simulink model "battery_sim"  (R2022a)
settings: Solver=VariableStepAuto  StartTime=0.0  StopTime=4000  RelTol=1e-3
undefined symbols (not defined in the file): T_AMB
libraries: fl_lib x13, nesl_utility x1
settings Model: DataDictionary=battery.sldd  Creator=Cristobal  LastModifiedBy=Cristobal
settings SFSimCC: SimTargetLang=C++  GPUAcceleration=on  SimDLTargetLibrary=cudnn

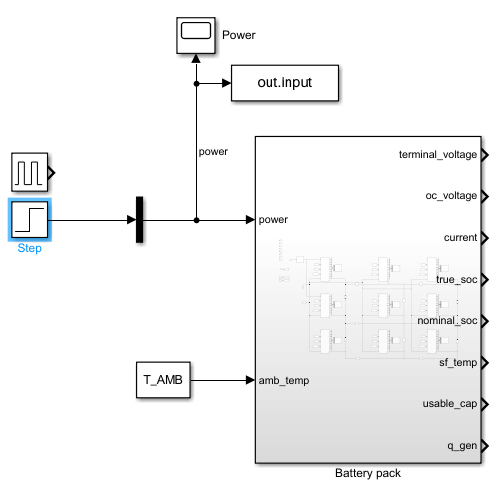
[thumbnail: Simulink's stored preview of the top-level diagram]
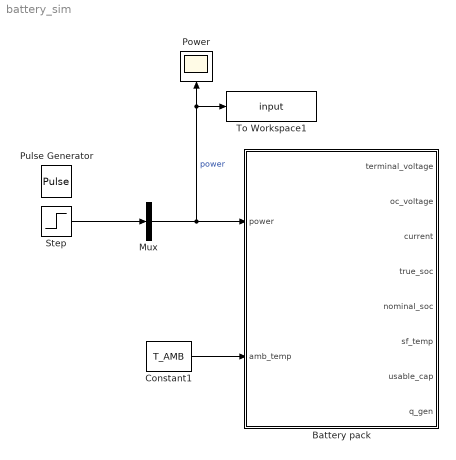
== system battery_sim ==
  Battery pack : Subsystem
  Constant1 : Constant  Value=T_AMB
  Mux : Mux  Inputs=1
  Power : Scope
  Pulse Generator : DiscretePulseGenerator  PulseType=Time based  Amplitude=1e-1  Period=300  PulseWidth=50
  Step : Step  Time=0  After=80  SampleTime=0
  To Workspace1 : ToWorkspace  VariableName=input  SaveFormat=Timeseries  SampleTime=-1
  wires:
  Constant1/1 -> Battery pack/2(amb_temp)
  Mux/1 -> To Workspace1/1, Power/1, Battery pack/1(power)  "power"
  Step/1 -> Mux/1

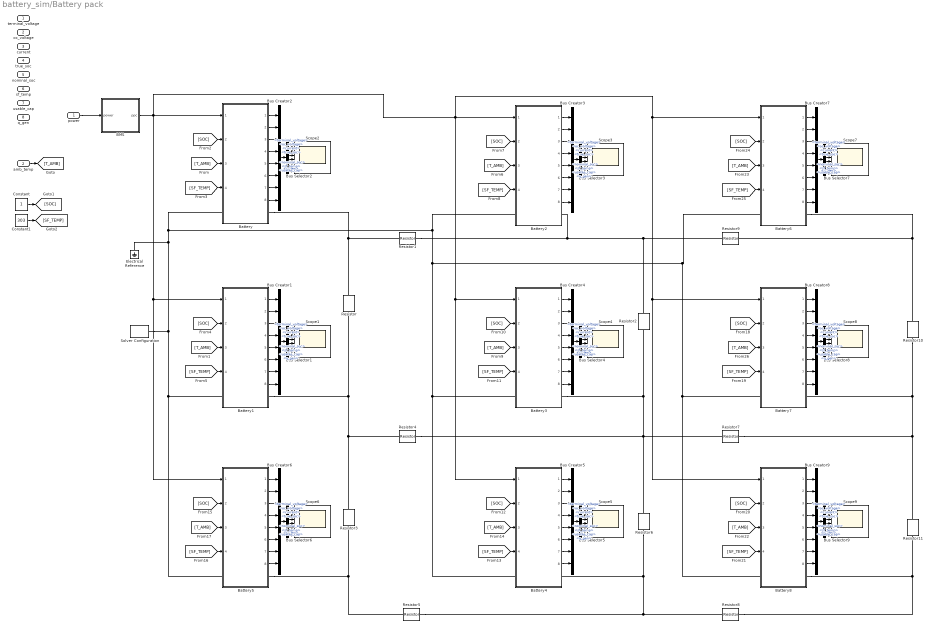
== system battery_sim/Battery pack ==
  power : Inport
  amb_temp : Inport  Port=2
  BMS : Subsystem  mask{Outputs=9}
      mask init:
      | % for i = 1:Outputs
      |     %     replace_block(gcb, "Name", "Terminator" + i, "Outport", "noprompt");
      |     % end
      |     % for i = Outputs + 1:64
      |     %     replace_block(gcb, "Name", "Terminator" + i, "Terminator", "noprompt");
      |     % end
      mask DialogControl DescGroupVar Prompt: BMS
      mask DialogControl DescTextVar Prompt: Ideal BMS that evenly distributes power
  Battery{,1..8} (9 alike) : Subsystem  ReferencedSubsystem=battery
  Bus Creator{1..9} (9 alike) : BusCreator  Inputs=8
  Bus Selector{1..9} (9 alike) : BusSelector  OutputSignals=terminal_voltage,oc_voltage,current,true_soc,nominal_soc,sf_temp,usable_cap,q_gen
  Constant : Constant
  Constant1 : Constant  Value=303
  Electrical Reference : fl_lib/Electrical/Electrical Elements/Electrical Reference
      settings: SourceProductBaseCode=PW,SS,VE
  Resistor{,1..11} (12 alike) : fl_lib/Electrical/Electrical Elements/Resistor  R=1e12 Ohm  i_specify=off  i_priority=None  i=0 A  i_nominal_specify=off  i_nominal_unit=A  i_nominal_value=1  v_specify=off  v_priority=None  v=0 V  v_nominal_specify=off  v_nominal_unit=V  v_nominal_value=1
      settings: SourceProductBaseCode=PW,SS,VE
  Scope{1..9} (9 alike) : Scope  NumInputPorts=8
  Solver Configuration : nesl_utility/Solver Configuration  PhysicalDomain=network_engine_domain  SubClassName=solver  LeftPortType=input  RightPortType=generic  Tones=[]  Harmonics=[]  SimulateNoise=off  Profile=off  UseLocalSampling=off  EnableSwitchedLinearOptims=on  FrequencyDomain=off  UseCCode=off  RelTol=0.001  AbsTol=0.001  MinStep=1e-09  ToWorkspace=off  RevertToSquareIcSolve=off  NumHomotopyIterations=100  PhasorMode=off  PhasorModeNumHarmonics=1  IndexReductionMethod=DerivativeReplacement  DoDC=off  ResidualTolerance=1e-09  UseLocalSolver=off  LocalSolverChoice=NE_BACKWARD_EULER_ADVANCER  LocalSolverSampleTime=0.001  DoFixedCost=off  MaxNonlinIter=3  MaxModeIter=2  ComputeImpulses=off  ImpulseIterations=2  LinearAlgebra=auto  LinearAlgebraNumThread=0  EquationFormulation=NE_TIME_EF  DelaysMemoryBudget=1024  AutomaticFiltering=on  FilteringTimeConstant=0.001  PartitionStorageMethod=AS_NEEDED  PartitionMemoryBudget=1024  PartitionMethod=ROBUST
      settings: SourceProductBaseCode=SS,PW,VE
  terminal_voltage : Outport
  oc_voltage : Outport  Port=2
  current : Outport  Port=3
  true_soc : Outport  Port=4
  nominal_soc : Outport  Port=5
  sf_temp : Outport  Port=6
  usable_cap : Outport  Port=7
  q_gen : Outport  Port=8
  wires:
  Bus Selector1/1 -> Scope1/1  "<terminal_voltage>"
  Bus Selector1/6 -> Scope1/6  "<sf_temp>"
  Bus Selector1/7 -> Scope1/7  "<usable_cap>"
  Bus Selector1/3 -> Scope1/3  "<current>"
  Bus Selector1/5 -> Scope1/5  "<nominal_soc>"
  Bus Selector1/2 -> Scope1/2  "<oc_voltage>"
  Bus Selector1/4 -> Scope1/4  "<true_soc>"
  Bus Selector1/8 -> Scope1/8  "<q_gen>"
  Battery1/1 -> Bus Creator1/1
  Battery1/2 -> Bus Creator1/2
  Battery1/3 -> Bus Creator1/3
  Battery1/4 -> Bus Creator1/4
  Battery1/5 -> Bus Creator1/5
  Battery1/6 -> Bus Creator1/6
  Battery1/7 -> Bus Creator1/7
  Battery1/8 -> Bus Creator1/8
  Bus Creator1/1 -> Bus Selector1/1
  amb_temp/1 -> [T_AMB]
  [T_AMB] -> Battery/3
  Constant/1 -> [SOC]
  Constant1/1 -> [SF_TEMP]
  [SOC] -> Battery/2
  [SF_TEMP] -> Battery/4
  [SOC] -> Battery1/2
  [T_AMB] -> Battery1/3
  [SF_TEMP] -> Battery1/4
  power/1 -> BMS/1(power)
  BMS/1(ppc) -> Battery8/1, Battery7/1, Battery6/1, Battery4/1, Battery3/1, Battery2/1, Battery1/1, Battery5/1, Battery/1
  Bus Creator2/1 -> Bus Selector2/1
  Bus Selector2/8 -> Scope2/8  "<q_gen>"
  Bus Selector2/4 -> Scope2/4  "<true_soc>"
  Bus Selector2/2 -> Scope2/2  "<oc_voltage>"
  Bus Selector2/5 -> Scope2/5  "<nominal_soc>"
  Bus Selector2/3 -> Scope2/3  "<current>"
  Bus Selector2/7 -> Scope2/7  "<usable_cap>"
  Bus Selector2/6 -> Scope2/6  "<sf_temp>"
  Bus Selector2/1 -> Scope2/1  "<terminal_voltage>"
  Battery/1 -> Bus Creator2/1
  Battery/2 -> Bus Creator2/2
  Battery/3 -> Bus Creator2/3
  Battery/4 -> Bus Creator2/4
  Battery/5 -> Bus Creator2/5
  Battery/6 -> Bus Creator2/6
  Battery/7 -> Bus Creator2/7
  Battery/8 -> Bus Creator2/8
  Battery2/8 -> Bus Creator3/8
  Battery2/7 -> Bus Creator3/7
  Battery2/6 -> Bus Creator3/6
  Battery2/5 -> Bus Creator3/5
  Battery2/4 -> Bus Creator3/4
  Battery2/3 -> Bus Creator3/3
  Battery2/2 -> Bus Creator3/2
  Battery2/1 -> Bus Creator3/1
  Bus Selector3/1 -> Scope3/1  "<terminal_voltage>"
  Bus Selector3/6 -> Scope3/6  "<sf_temp>"
  Bus Selector3/7 -> Scope3/7  "<usable_cap>"
  Bus Selector3/3 -> Scope3/3  "<current>"
  Bus Selector3/5 -> Scope3/5  "<nominal_soc>"
  Bus Selector3/2 -> Scope3/2  "<oc_voltage>"
  Bus Selector3/4 -> Scope3/4  "<true_soc>"
  Bus Selector3/8 -> Scope3/8  "<q_gen>"
  Bus Creator3/1 -> Bus Selector3/1
  [SF_TEMP] -> Battery2/4
  [SOC] -> Battery2/2
  [T_AMB] -> Battery2/3
  [T_AMB] -> Battery3/3
  [SOC] -> Battery3/2
  [SF_TEMP] -> Battery3/4
  Bus Creator4/1 -> Bus Selector4/1
  Bus Selector4/8 -> Scope4/8  "<q_gen>"
  Bus Selector4/4 -> Scope4/4  "<true_soc>"
  Bus Selector4/2 -> Scope4/2  "<oc_voltage>"
  Bus Selector4/5 -> Scope4/5  "<nominal_soc>"
  Bus Selector4/3 -> Scope4/3  "<current>"
  Bus Selector4/7 -> Scope4/7  "<usable_cap>"
  Bus Selector4/6 -> Scope4/6  "<sf_temp>"
  Bus Selector4/1 -> Scope4/1  "<terminal_voltage>"
  Battery3/1 -> Bus Creator4/1
  Battery3/2 -> Bus Creator4/2
  Battery3/3 -> Bus Creator4/3
  Battery3/4 -> Bus Creator4/4
  Battery3/5 -> Bus Creator4/5
  Battery3/6 -> Bus Creator4/6
  Battery3/7 -> Bus Creator4/7
  Battery3/8 -> Bus Creator4/8
  Battery4/8 -> Bus Creator5/8
  Battery4/7 -> Bus Creator5/7
  Battery4/6 -> Bus Creator5/6
  Battery4/5 -> Bus Creator5/5
  Battery4/4 -> Bus Creator5/4
  Battery4/3 -> Bus Creator5/3
  Battery4/2 -> Bus Creator5/2
  Battery4/1 -> Bus Creator5/1
  Bus Selector5/1 -> Scope5/1  "<terminal_voltage>"
  Bus Selector5/6 -> Scope5/6  "<sf_temp>"
  Bus Selector5/7 -> Scope5/7  "<usable_cap>"
  Bus Selector5/3 -> Scope5/3  "<current>"
  Bus Selector5/5 -> Scope5/5  "<nominal_soc>"
  Bus Selector5/2 -> Scope5/2  "<oc_voltage>"
  Bus Selector5/4 -> Scope5/4  "<true_soc>"
  Bus Selector5/8 -> Scope5/8  "<q_gen>"
  Bus Creator5/1 -> Bus Selector5/1
  [SF_TEMP] -> Battery4/4
  [SOC] -> Battery4/2
  [T_AMB] -> Battery4/3
  [T_AMB] -> Battery5/3
  [SOC] -> Battery5/2
  [SF_TEMP] -> Battery5/4
  Bus Creator6/1 -> Bus Selector6/1
  Bus Selector6/8 -> Scope6/8  "<q_gen>"
  Bus Selector6/4 -> Scope6/4  "<true_soc>"
  Bus Selector6/2 -> Scope6/2  "<oc_voltage>"
  Bus Selector6/5 -> Scope6/5  "<nominal_soc>"
  Bus Selector6/3 -> Scope6/3  "<current>"
  Bus Selector6/7 -> Scope6/7  "<usable_cap>"
  Bus Selector6/6 -> Scope6/6  "<sf_temp>"
  Bus Selector6/1 -> Scope6/1  "<terminal_voltage>"
  Battery5/1 -> Bus Creator6/1
  Battery5/2 -> Bus Creator6/2
  Battery5/3 -> Bus Creator6/3
  Battery5/4 -> Bus Creator6/4
  Battery5/5 -> Bus Creator6/5
  Battery5/6 -> Bus Creator6/6
  Battery5/7 -> Bus Creator6/7
  Battery5/8 -> Bus Creator6/8
  [T_AMB] -> Battery8/3
  [SOC] -> Battery8/2
  [SF_TEMP] -> Battery8/4
  Bus Creator9/1 -> Bus Selector9/1
  Bus Selector9/8 -> Scope9/8  "<q_gen>"
  Bus Selector9/4 -> Scope9/4  "<true_soc>"
  Bus Selector9/2 -> Scope9/2  "<oc_voltage>"
  Bus Selector9/5 -> Scope9/5  "<nominal_soc>"
  Bus Selector9/3 -> Scope9/3  "<current>"
  Bus Selector9/7 -> Scope9/7  "<usable_cap>"
  Bus Selector9/6 -> Scope9/6  "<sf_temp>"
  Bus Selector9/1 -> Scope9/1  "<terminal_voltage>"
  Battery8/1 -> Bus Creator9/1
  Battery8/2 -> Bus Creator9/2
  Battery8/3 -> Bus Creator9/3
  Battery8/4 -> Bus Creator9/4
  Battery8/5 -> Bus Creator9/5
  Battery8/6 -> Bus Creator9/6
  Battery8/7 -> Bus Creator9/7
  Battery8/8 -> Bus Creator9/8
  Battery7/8 -> Bus Creator8/8
  Battery7/7 -> Bus Creator8/7
  Battery7/6 -> Bus Creator8/6
  Battery7/5 -> Bus Creator8/5
  Battery7/4 -> Bus Creator8/4
  Battery7/3 -> Bus Creator8/3
  Battery7/2 -> Bus Creator8/2
  Battery7/1 -> Bus Creator8/1
  Bus Selector8/1 -> Scope8/1  "<terminal_voltage>"
  Bus Selector8/6 -> Scope8/6  "<sf_temp>"
  Bus Selector8/7 -> Scope8/7  "<usable_cap>"
  Bus Selector8/3 -> Scope8/3  "<current>"
  Bus Selector8/5 -> Scope8/5  "<nominal_soc>"
  Bus Selector8/2 -> Scope8/2  "<oc_voltage>"
  Bus Selector8/4 -> Scope8/4  "<true_soc>"
  Bus Selector8/8 -> Scope8/8  "<q_gen>"
  Bus Creator8/1 -> Bus Selector8/1
  [SF_TEMP] -> Battery7/4
  [SOC] -> Battery7/2
  [T_AMB] -> Battery7/3
  [T_AMB] -> Battery6/3
  [SOC] -> Battery6/2
  [SF_TEMP] -> Battery6/4
  Bus Creator7/1 -> Bus Selector7/1
  Bus Selector7/8 -> Scope7/8  "<q_gen>"
  Bus Selector7/4 -> Scope7/4  "<true_soc>"
  Bus Selector7/2 -> Scope7/2  "<oc_voltage>"
  Bus Selector7/5 -> Scope7/5  "<nominal_soc>"
  Bus Selector7/3 -> Scope7/3  "<current>"
  Bus Selector7/7 -> Scope7/7  "<usable_cap>"
  Bus Selector7/6 -> Scope7/6  "<sf_temp>"
  Bus Selector7/1 -> Scope7/1  "<terminal_voltage>"
  Battery6/1 -> Bus Creator7/1
  Battery6/2 -> Bus Creator7/2
  Battery6/3 -> Bus Creator7/3
  Battery6/4 -> Bus Creator7/4
  Battery6/5 -> Bus Creator7/5
  Battery6/6 -> Bus Creator7/6
  Battery6/7 -> Bus Creator7/7
  Battery6/8 -> Bus Creator7/8
  connections:
  Battery/RConn1 -- Resistor1/RConn1 -- Resistor/LConn1
  Battery1/LConn1 -- Battery5/LConn1 -- Solver Configuration/RConn1 -- Battery8/LConn1 -- Battery7/LConn1 -- Battery6/LConn1 -- Battery4/LConn1 -- Battery3/LConn1 -- Battery2/LConn1 -- Battery/LConn1 -- Electrical Reference/LConn1
  Battery1/RConn1 -- Resistor4/RConn1 -- Resistor3/LConn1 -- Resistor/RConn1
  Resistor1/LConn1 -- Resistor9/RConn1 -- Resistor2/LConn1 -- Battery2/RConn1
  Battery3/RConn1 -- Resistor7/RConn1 -- Resistor6/LConn1 -- Resistor4/LConn1 -- Resistor2/RConn1
  Battery5/RConn1 -- Resistor3/RConn1 -- Resistor5/RConn1
  Resistor5/LConn1 -- Resistor8/RConn1 -- Resistor6/RConn1 -- Battery4/RConn1
  Resistor8/LConn1 -- Battery8/RConn1 -- Resistor11/RConn1
  Resistor11/LConn1 -- Resistor7/LConn1 -- Resistor10/RConn1 -- Battery7/RConn1
  Resistor10/LConn1 -- Battery6/RConn1 -- Resistor9/LConn1

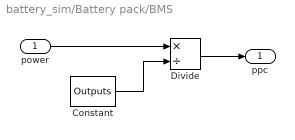
== system battery_sim/Battery pack/BMS ==
  power : Inport
  Constant : Constant  Value=Outputs
  Divide : Product  Inputs=*/
  ppc : Outport
  wires:
  Constant/1 -> Divide/2
  power/1 -> Divide/1
  Divide/1 -> ppc/1
